simulink model "lab2"  (R2020b)
settings: Solver=VariableStepAuto  StartTime=0.0  StopTime=100  RelTol=1e-3
values from neighbouring files (symbols this model uses):
  b = 500    [values.m]
  k1 = 300    [values.m]
  k2 = 2000    [values.m]
  m1 = 10000    [values.m]
  m2 = 50    [values.m]
settings Model: OrderedModelArguments=off  Creator=sushma  LastModifiedBy=sushma

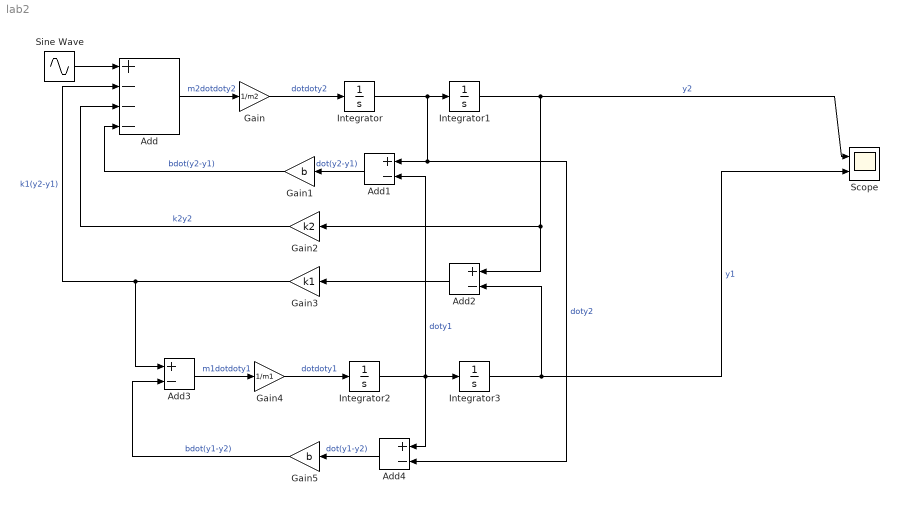
== system lab2 ==
  Add : Sum  Inputs=+---
  Add{1..4} (4 alike) : Sum  Inputs=+-
  Gain : Gain  Gain=1/m2
  Gain1 : Gain  Gain=b
  Gain2 : Gain  Gain=k2
  Gain3 : Gain  Gain=k1
  Gain4 : Gain  Gain=1/m1
  Gain5 : Gain  Gain=b
  Integrator{,1..3} (4 alike) : Integrator
  Scope : Scope  NumInputPorts=2
  Sine Wave : Sin  SampleTime=0
  wires:
  Add/1 -> Gain/1  "m2dotdoty2"
  Gain/1 -> Integrator/1  "dotdoty2"
  Integrator/1 -> Add4/2, Add1/1, Integrator1/1  "doty2"
  Integrator2/1 -> Add4/1, Add1/2, Integrator3/1  "doty1"
  Gain4/1 -> Integrator2/1  "dotdoty1"
  Add3/1 -> Gain4/1  "m1dotdoty1"
  Add1/1 -> Gain1/1  "dot(y2-y1)"
  Add2/1 -> Gain3/1
  Integrator3/1 -> Scope/2, Add2/2  "y1"
  Integrator1/1 -> Gain2/1, Add2/1, Scope/1  "y2"
  Add4/1 -> Gain5/1  "dot(y1-y2)"
  Gain5/1 -> Add3/2  "bdot(y1-y2)"
  Gain1/1 -> Add/4  "bdot(y2-y1)"
  Gain2/1 -> Add/3  "k2y2"
  Gain3/1 -> Add3/1, Add/2  "k1(y2-y1)"
  Sine Wave/1 -> Add/1
